simulink model "Model_Simulink"  (Simulink 7.6)
settings: Solver=ode3  StartTime=0.0  StopTime=4800  FixedStep=1  RelTol=1e-3
libraries: simulink x3, dspsrcs4 x2
settings Model: Creator=skener  LastModifiedBy=Admin

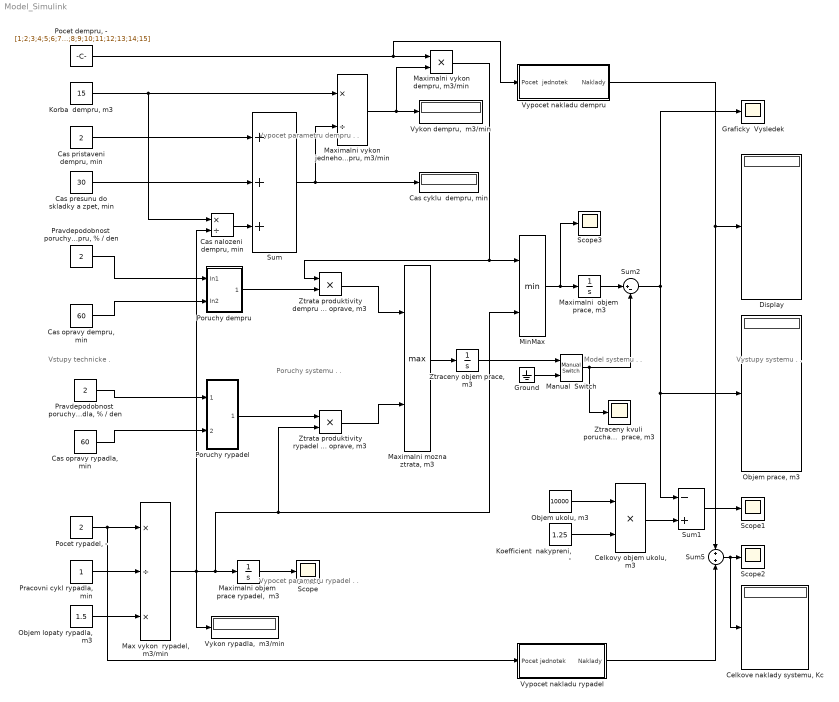
== system Model_Simulink ==
  note: Vstupy technicke
      |
      |
      |
      |
      |
      |
      |
      |
      |
      |
      |
      |
      |
      |
      |
      |
      |
      |
      |
      |
      |
      |
      |
      |
      |
      |
      |
      |
      |
      |
      |
      |
      |
      |
      |
      |
      |
      |
      |
      |
      |
      |
      |
      |
      |
      |
      |
      |
      |
      |
      |
      |
      |
      |
      |
      |
      |
      | .
  note: Vystupy systemu     .
      |
      |
      |
      |
      |
      |
      |
      |
      |
      |
      |
      |
      |
      |
      |
      |
      |
      |
      |
      |
      |
      |
      |
      |
      |
      |
      |
      |
      |
      |
      |
      |
      |
      |
      |
      |
      |
      |
      |
      |
      |
      |
      |
      |
      |
      |
      |
      |
      |
      |
      |
      |
      |
      |
      |
      |
      |
      | .
  note: Model systemu                                                              .
      |
      |
      |
      |
      |
      |
      |
      |
      |
      |
      |
      |
      |
      |
      |
      |
      |
      |
      |
      |
      |
      |
      |
      |
      |
      |
      |
      |
      |
      |
      |
      |
      |
      |
      |
      |
      |
      |
      |
      |
      |
      |
      |
      |
      |
      |
      |
      |
      |
      |
      |
      |
      |
      |
      |
      |
      |
      | .
  note: Vypocet parametru dempru                                                                                                                   .
      |
      |
      |
      |
      |
      |
      |
      |
      |
      |
      |
      |
      |
      |
      |
      |
      |
      |
      | .
  note: Vypocet parametru rypadel                                                                                                                    .
      |
      |
      |
      |
      |
      |
      |
      |
      |
      |
      |
      |
      |
      |
      |
      |
      | .
  note: Poruchy systemu                                                                                                                                       .
      |
      |
      |
      |
      |
      |
      |
      |
      |
      |
      |
      |
      |
      |
      |
      |
      |
      |
      | .
  "Cas cyklu  dempru, min" : Display
  "Cas nalozeni  dempru, min" : Product  Inputs=*/  RndMeth=Zero
  "Cas opravy dempru, min" : Constant  Value=60
  "Cas opravy rypadla, min" : Constant  Value=60
  "Cas presunu do skladky a zpet, min" : Constant  Value=30
  "Cas pristaveni dempru, min" : Constant  Value=2
  "Celkove naklady systemu, Kc" : Display
      settings: Format=bank
  "Celkovy objem ukolu, m3" : Product  RndMeth=Zero
  Display : Display
      settings: Format=bank
  Graficky  Vysledek : Scope
  Ground : Ground
  "Koefficient  nakypreni, -" : Constant  Value=1.25
  "Korba  dempru, m3" : Constant  Value=15
  Manual  Switch : simulink/Signal Routing/Manual Switch  SystemSampleTime=-1  sw=1  action=0  varsize=off
  "Max vykon  rypadel, m3/min" : Product  Inputs=*/*  RndMeth=Zero
  "Maximalni  objem  prace, m3" : Integrator
  "Maximalni mozna ztrata, m3" : MinMax  Function=max  Inputs=2
  "Maximalni objem  prace rypadel,  m3" : Integrator
  "Maximalni vykon dempru, m3/min" : Product  RndMeth=Zero
  "Maximalni vykon jedneho dempru, m3/min" : Product  Inputs=*/  RndMeth=Zero
  MinMax : MinMax  Inputs=2
  "Objem lopaty rypadla, m3" : Constant  Value=1.5
  "Objem prace, m3" : Display
      settings: Format=bank
  "Objem ukolu, m3" : Constant  Value=10000
  "Pocet dempru, -" : Constant  Value=[1;2;3;4;5;6;7;8;9;10;11;12;13;14;15]
  "Pocet rypadel, -" : Constant  Value=2
  Poruchy dempru : Subsystem
  Poruchy rypadel : Subsystem
  "Pracovni cykl rypadla, min" : Constant
  "Pravdepodobnost  poruchy dempru, % / den" : Constant  Value=2
  "Pravdepodobnost  poruchy rypadla, % / den" : Constant  Value=2
  Scope{,1..3} (4 alike) : Scope
      Scope1 settings: SaveName=ScopeData2
      Scope2 settings: SaveName=ScopeData9
      Scope3 settings: SaveName=ScopeData6
  Sum : Sum  Inputs=+++
  Sum1 : Sum  Inputs=-+
  Sum2 : Sum  Inputs=|+-
  Sum5 : Sum  Inputs=+|+
  "Vykon dempru,  m3/min" : Display
  "Vykon rypadla,  m3/min" : Display
  Vypocet nakladu dempru : Subsystem
  Vypocet nakladu rypadel : Subsystem
  "Ztraceny kvuli  porucham objem  prace, m3" : Scope
      settings: SaveName=ScopeData5
  "Ztraceny objem prace, m3" : Integrator
  "Ztrata produktivity dempru kvuli oprave, m3" : Product  RndMeth=Zero
  "Ztrata produktivity rypadel kvuli oprave, m3" : Product  RndMeth=Zero
  wires:
  "Cas pristaveni dempru, min"/1 -> Sum/1
  "Cas presunu do skladky a zpet, min"/1 -> Sum/2
  "Korba  dempru, m3"/1 -> "Maximalni vykon jedneho dempru, m3/min"/1, "Cas nalozeni  dempru, min"/1
  "Pocet rypadel, -"/1 -> "Max vykon  rypadel, m3/min"/1, Vypocet nakladu rypadel/1(Pocet jednotek)
  "Objem lopaty rypadla, m3"/1 -> "Max vykon  rypadel, m3/min"/3
  "Cas nalozeni  dempru, min"/1 -> Sum/3
  Sum/1 -> "Maximalni vykon jedneho dempru, m3/min"/2, "Cas cyklu  dempru, min"/1
  "Pocet dempru, -"/1 -> "Maximalni vykon dempru, m3/min"/1, Vypocet nakladu dempru/1(Pocet  jednotek)
  "Maximalni vykon jedneho dempru, m3/min"/1 -> "Maximalni vykon dempru, m3/min"/2, "Vykon dempru,  m3/min"/1
  "Maximalni  objem  prace, m3"/1 -> Sum2/1
  "Max vykon  rypadel, m3/min"/1 -> "Cas nalozeni  dempru, min"/2, "Vykon rypadla,  m3/min"/1, "Maximalni objem  prace rypadel,  m3"/1, MinMax/2, "Ztrata produktivity rypadel kvuli oprave, m3"/2
  "Maximalni objem  prace rypadel,  m3"/1 -> Scope/1
  MinMax/1 -> "Maximalni  objem  prace, m3"/1, Scope3/1
  "Maximalni vykon dempru, m3/min"/1 -> "Ztrata produktivity dempru kvuli oprave, m3"/1, MinMax/1
  "Objem ukolu, m3"/1 -> "Celkovy objem ukolu, m3"/1
  "Koefficient  nakypreni, -"/1 -> "Celkovy objem ukolu, m3"/2
  "Celkovy objem ukolu, m3"/1 -> Sum1/2
  Sum1/1 -> Scope1/1
  "Pravdepodobnost  poruchy dempru, % / den"/1 -> Poruchy dempru/1(In1)
  "Cas opravy dempru, min"/1 -> Poruchy dempru/2(In2)
  "Pravdepodobnost  poruchy rypadla, % / den"/1 -> Poruchy rypadel/1(In1)
  "Cas opravy rypadla, min"/1 -> Poruchy rypadel/2(In2)
  "Pracovni cykl rypadla, min"/1 -> "Max vykon  rypadel, m3/min"/2
  Poruchy dempru/1(Opravy) -> "Ztrata produktivity dempru kvuli oprave, m3"/2
  Poruchy rypadel/1(Opravy) -> "Ztrata produktivity rypadel kvuli oprave, m3"/1
  "Ztrata produktivity dempru kvuli oprave, m3"/1 -> "Maximalni mozna ztrata, m3"/1
  "Ztrata produktivity rypadel kvuli oprave, m3"/1 -> "Maximalni mozna ztrata, m3"/2
  Sum2/1 -> Graficky  Vysledek/1, Sum1/1, "Objem prace, m3"/1
  Ground/1 -> Manual  Switch/2
  "Maximalni mozna ztrata, m3"/1 -> "Ztraceny objem prace, m3"/1
  "Ztraceny objem prace, m3"/1 -> Manual  Switch/1
  Manual  Switch/1 -> Sum2/2, "Ztraceny kvuli  porucham objem  prace, m3"/1
  Vypocet nakladu dempru/1(Naklady) -> Display/1, Sum5/1
  Vypocet nakladu rypadel/1(Naklady) -> Sum5/2
  Sum5/1 -> "Celkove naklady systemu, Kc"/1, Scope2/1

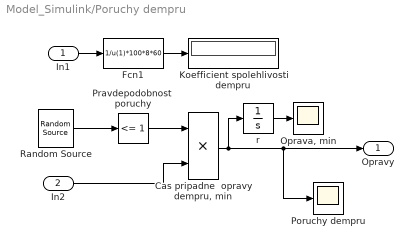
== system Model_Simulink/Poruchy dempru ==
  In1 : Inport
  In2 : Inport  Port=2
  "Cas pripadne  opravy dempru, min" : Product  RndMeth=Zero
  Fcn1 : Fcn  Expr=1/u(1)*100*8*60
  Koefficient spolehlivosti dempru : Display
      settings: Format=bank
  "Oprava, min" : Scope
      settings: SaveName=ScopeData4
  Poruchy dempru : Scope
      settings: SaveName=ScopeData3
  Pravdepodobnost  poruchy : simulink/Logic and Bit Operations/Compare To Constant  SystemSampleTime=-1  relop=<=  const=1  LogicOutDataTypeMode=boolean
  Random Source : dspsrcs4/Random Source  SrcType=Uniform  NormMethod=Ziggurat  CltLength=12  MinVal=[0;0;0;0;0;0;0;0;0;0;0;0;0;0;0]  MaxVal=[24000;12000;8000;6000;4800;4000;3428;3000;2666;2400;2181;2000;1846;1714;1600]  MeanVal=0  VarVal=1  RepMode=Not repeatable  rawSeed=1  IsInherit=off  SampMode=Discrete  SampTime=1  SampFrame=1  DataType=Double  OutComplex=Real
  r : Integrator
  Opravy : Outport
  wires:
  Fcn1/1 -> Koefficient spolehlivosti dempru/1
  Random Source/1 -> Pravdepodobnost  poruchy/1
  Pravdepodobnost  poruchy/1 -> "Cas pripadne  opravy dempru, min"/1
  "Cas pripadne  opravy dempru, min"/1 -> Poruchy dempru/1, Opravy/1, r/1
  r/1 -> "Oprava, min"/1
  In1/1 -> Fcn1/1
  In2/1 -> "Cas pripadne  opravy dempru, min"/2

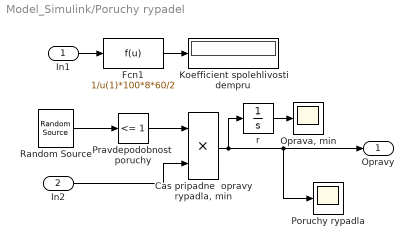
== system Model_Simulink/Poruchy rypadel ==
  In1 : Inport
  In2 : Inport  Port=2
  "Cas pripadne  opravy rypadla, min" : Product  RndMeth=Zero
  Fcn1 : Fcn  Expr=1/u(1)*100*8*60/2
  Koefficient spolehlivosti dempru : Display
      settings: Format=bank
  "Oprava, min" : Scope
      settings: SaveName=ScopeData4
  Poruchy rypadla : Scope
      settings: SaveName=ScopeData3
  Pravdepodobnost  poruchy : simulink/Logic and Bit Operations/Compare To Constant  SystemSampleTime=-1  relop=<=  const=1  LogicOutDataTypeMode=boolean
  Random Source : dspsrcs4/Random Source  SrcType=Uniform  NormMethod=Ziggurat  CltLength=12  MinVal=0  MaxVal=12000  MeanVal=0  VarVal=1  RepMode=Not repeatable  rawSeed=1  IsInherit=off  SampMode=Discrete  SampTime=1  SampFrame=1  DataType=Double  OutComplex=Real
  r : Integrator
  Opravy : Outport
  wires:
  Fcn1/1 -> Koefficient spolehlivosti dempru/1
  Random Source/1 -> Pravdepodobnost  poruchy/1
  Pravdepodobnost  poruchy/1 -> "Cas pripadne  opravy rypadla, min"/1
  "Cas pripadne  opravy rypadla, min"/1 -> Poruchy rypadla/1, Opravy/1, r/1
  r/1 -> "Oprava, min"/1
  In1/1 -> Fcn1/1
  In2/1 -> "Cas pripadne  opravy rypadla, min"/2

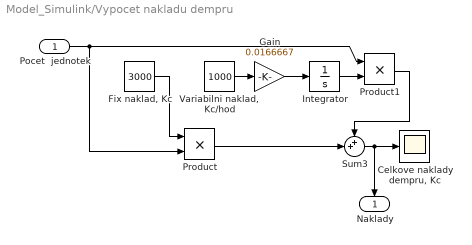
== system Model_Simulink/Vypocet nakladu dempru ==
  Pocet  jednotek : Inport
  "Celkove naklady dempru, Kc" : Scope
      settings: SaveName=ScopeData7
  "Fix naklad, Kc" : Constant  Value=3000
  Gain : Gain  Gain=0.0166667
  Integrator : Integrator
  Product : Product  RndMeth=Zero
  Product1 : Product  RndMeth=Zero
  Sum3 : Sum  Inputs=++|
  "Variabilni naklad,  Kc/hod" : Constant  Value=1000
  Naklady : Outport
  wires:
  "Fix naklad, Kc"/1 -> Product/1
  Product/1 -> Sum3/2
  "Variabilni naklad,  Kc/hod"/1 -> Gain/1
  Gain/1 -> Integrator/1
  Sum3/1 -> "Celkove naklady dempru, Kc"/1, Naklady/1
  Integrator/1 -> Product1/2
  Product1/1 -> Sum3/1
  Pocet  jednotek/1 -> Product/2, Product1/1

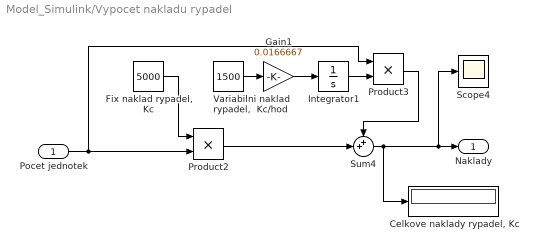
== system Model_Simulink/Vypocet nakladu rypadel ==
  Pocet jednotek : Inport
  "Celkove naklady rypadel, Kc" : Display
      settings: Format=bank
  "Fix naklad rypadel, Kc" : Constant  Value=5000
  Gain1 : Gain  Gain=0.0166667
  Integrator1 : Integrator
  Product2 : Product  RndMeth=Zero
  Product3 : Product  RndMeth=Zero
  Scope4 : Scope
      settings: SaveName=ScopeData8
  Sum4 : Sum  Inputs=++|
  "Variabilni naklad rypadel,  Kc/hod" : Constant  Value=1500
  Naklady : Outport
  wires:
  "Fix naklad rypadel, Kc"/1 -> Product2/1
  Product2/1 -> Sum4/2
  "Variabilni naklad rypadel,  Kc/hod"/1 -> Gain1/1
  Gain1/1 -> Integrator1/1
  Sum4/1 -> "Celkove naklady rypadel, Kc"/1, Scope4/1, Naklady/1
  Integrator1/1 -> Product3/2
  Product3/1 -> Sum4/1
  Pocet jednotek/1 -> Product2/2, Product3/1
